simulink model "tekniska"  (R2018a)
settings: Solver=VariableStepAuto  StartTime=0.0  StopTime=3600  RelTol=1e-3
undefined symbols (not defined in the file): m, n
libraries: simulink x1
settings Model: Creator=wass  LastModifiedBy=wass

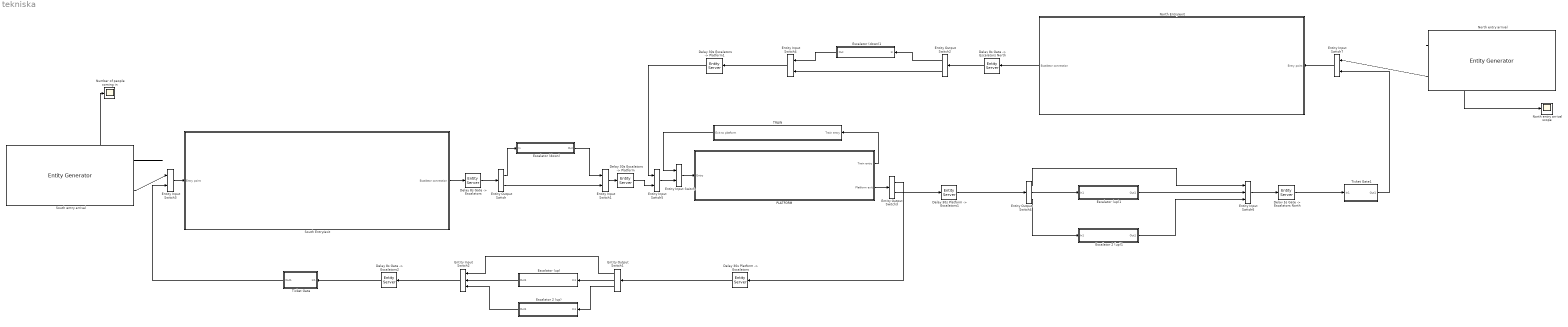
== system tekniska ==
  "Delay 30s Escalators -> Platform" : EntityServer  InputPortMessageModes=m  OutputPortMessageModes=m  Capacity=inf  ServiceTimeValue=30
  "Delay 30s Escalators -> Platform1" : EntityServer  InputPortMessageModes=m  OutputPortMessageModes=m  Capacity=inf  ServiceTimeValue=30
  "Delay 30s Platform -> Escalators" : EntityServer  InputPortMessageModes=m  OutputPortMessageModes=m  Capacity=inf  ServiceTimeValue=30
  "Delay 30s Platform -> Escalators1" : EntityServer  InputPortMessageModes=m  OutputPortMessageModes=m  Capacity=inf  ServiceTimeValue=30
  "Delay 5s Gate -> Escalators North" : EntityServer  InputPortMessageModes=m  OutputPortMessageModes=m  Capacity=inf  ServiceTimeValue=5
  "Delay 8s Gate -> Escalators" : EntityServer  InputPortMessageModes=m  OutputPortMessageModes=m  Capacity=inf  ServiceTimeValue=8
  "Delay 8s Gate -> Escalators North " : EntityServer  InputPortMessageModes=m  OutputPortMessageModes=m  Capacity=inf  ServiceTimeValue=5
  "Delay 8s Gate -> Escalators2" : EntityServer  InputPortMessageModes=m  OutputPortMessageModes=m  Capacity=inf  ServiceTimeValue=8
  Entity Input Switch{,1,3..5,7} (6 alike) : EntityInputSwitch  InputPortMessageModes=m,m  OutputPortMessageModes=m
  Entity Input Switch2 : EntityInputSwitch  InputPortMessageModes=m,m,m  OutputPortMessageModes=m  NumberInputPorts=3
      settings: InputPortMap=u1,u2,u3
  Entity Input Switch6 : EntityInputSwitch  InputPortMessageModes=m,m,m  OutputPortMessageModes=m  NumberInputPorts=3
      settings: InputPortMap=u1,u2,u3
  Entity Output Switch : EntityOutputSwitch  InputPortMessageModes=m  OutputPortMessageModes=m,m  SwitchingCriterion=Equiprobable  SwitchAttributeName=Attribute1
  Entity Output Switch1 : EntityOutputSwitch  InputPortMessageModes=m  OutputPortMessageModes=m,m,m  NumberOutputPorts=3  SwitchAttributeName=Attribute1
      settings: OutputPortMap=o0,o1,o2
  Entity Output Switch2 : EntityOutputSwitch  InputPortMessageModes=m  OutputPortMessageModes=m,m  SwitchingCriterion=Equiprobable  SwitchAttributeName=Attribute1
  Entity Output Switch3 : EntityOutputSwitch  InputPortMessageModes=m  OutputPortMessageModes=m,m  SwitchAttributeName=Attribute1
  Entity Output Switch4 : EntityOutputSwitch  InputPortMessageModes=m  OutputPortMessageModes=m,m,m  NumberOutputPorts=3  SwitchAttributeName=Attribute1
      settings: OutputPortMap=o0,o1,o2
  Escalator (down) : Subsystem
  Escalator (down)1 : Subsystem
  Escalator (up) : Subsystem
  Escalator (up)1 : Subsystem
  Escalator 2 (up) : Subsystem
  Escalator 2 (up)1 : Subsystem
  North Entry/exit : Subsystem
  North entry arrival : EntityGenerator  OutputPortMessageModes=n,m  TimeSource=MATLAB action  IntergenerationTimeAction=|  GenerateEntityAtSimulationStart=off  AttributeName=Incoming  AttributeInitialValue=2  NumberEntitiesDeparted=on  EntityType=Structured  EntityTypeName=Entity
      | wait_per_person = 10;
      | dt = exprnd(wait_per_person);
      settings: OutputPortMap=o0,o3
  North entry arrival scope : Scope
  Number of people coming in : Scope
  PLATFORM : Subsystem
  South Entry/exit : Subsystem
  South entry arrival : EntityGenerator  OutputPortMessageModes=n,m  TimeSource=MATLAB action  IntergenerationTimeAction=|  GenerateEntityAtSimulationStart=off  AttributeName=Incoming  AttributeInitialValue=2  NumberEntitiesDeparted=on  EntityType=Structured  EntityTypeName=Entity
      | wait_per_person = 5;
      | dt = exprnd(wait_per_person);
      settings: OutputPortMap=o0,o3
  TRAIN : Subsystem
  Ticket Gate : Subsystem
  Ticket Gate1 : Subsystem
  wires:
  TRAIN/1(Exit to platform) -> Entity Input Switch/1
  Escalator (up)/1(Out1) -> Entity Input Switch2/2
  Entity Input Switch/1 -> PLATFORM/1(Entry)
  South entry arrival/1 -> Number of people coming in/1
  Entity Output Switch1/3 -> Escalator 2 (up)/1(In1)
  PLATFORM/1(Train entry) -> TRAIN/1(Train entry)
  South Entry/exit/1(Escalator connection) -> "Delay 8s Gate -> Escalators"/1
  Escalator (down)/1(Out) -> Entity Input Switch1/1
  South entry arrival/2 -> Entity Input Switch3/1
  Entity Output Switch/1 -> Escalator (down)/1(In)
  Entity Output Switch1/2 -> Escalator (up)/1(In1)
  Entity Input Switch2/1 -> "Delay 8s Gate -> Escalators2"/1
  Entity Output Switch1/1 -> Entity Input Switch2/1
  Entity Input Switch1/1 -> "Delay 30s Escalators -> Platform"/1
  Escalator 2 (up)/1(Out1) -> Entity Input Switch2/3
  Entity Input Switch3/1 -> South Entry/exit/1(Entry point)
  Ticket Gate/1(Out1) -> Entity Input Switch3/2
  Entity Output Switch/2 -> Entity Input Switch1/2
  "Delay 8s Gate -> Escalators"/1 -> Entity Output Switch/1
  "Delay 8s Gate -> Escalators2"/1 -> Ticket Gate/1(In1)
  "Delay 30s Platform -> Escalators"/1 -> Entity Output Switch1/1
  Escalator (down)1/1(Out) -> Entity Input Switch4/1
  Entity Output Switch2/1 -> Escalator (down)1/1(In)
  Entity Output Switch2/2 -> Entity Input Switch4/2
  North Entry/exit/1(Escalator connection) -> "Delay 8s Gate -> Escalators North "/1
  "Delay 8s Gate -> Escalators North "/1 -> Entity Output Switch2/1
  Entity Input Switch4/1 -> "Delay 30s Escalators -> Platform1"/1
  "Delay 30s Escalators -> Platform"/1 -> Entity Input Switch5/2
  "Delay 30s Escalators -> Platform1"/1 -> Entity Input Switch5/1
  Entity Input Switch5/1 -> Entity Input Switch/2
  PLATFORM/2(Platform exit) -> Entity Output Switch3/1
  Entity Output Switch3/1 -> "Delay 30s Platform -> Escalators"/1
  Entity Output Switch3/2 -> "Delay 30s Platform -> Escalators1"/1
  Entity Input Switch6/1 -> "Delay 5s Gate -> Escalators North"/1
  Ticket Gate1/1(Out1) -> Entity Input Switch7/2
  Entity Output Switch4/2 -> Escalator (up)1/1(In1)
  Entity Output Switch4/3 -> Escalator 2 (up)1/1(In1)
  Escalator (up)1/1(Out1) -> Entity Input Switch6/2
  Escalator 2 (up)1/1(Out1) -> Entity Input Switch6/3
  Entity Output Switch4/1 -> Entity Input Switch6/1
  "Delay 30s Platform -> Escalators1"/1 -> Entity Output Switch4/1
  "Delay 5s Gate -> Escalators North"/1 -> Ticket Gate1/1(In1)
  Entity Input Switch7/1 -> North Entry/exit/1(Entry point)
  North entry arrival/1 -> North entry arrival scope/1
  North entry arrival/2 -> Entity Input Switch7/1

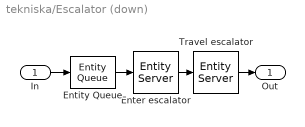
== system tekniska/Escalator (down) ==
  In : Inport
  Enter escalator : EntityServer  InputPortMessageModes=m  OutputPortMessageModes=m  Capacity=1  ServiceTimeValue=1
  Entity Queue : EntityQueue  InputPortMessageModes=m  OutputPortMessageModes=m  Capacity=inf
      settings: OutputPortMap=o5
  Travel escalator : EntityServer  InputPortMessageModes=m  OutputPortMessageModes=m  Capacity=inf  ServiceTimeValue=40
  Out : Outport
  wires:
  In/1 -> Entity Queue/1
  Enter escalator/1 -> Travel escalator/1
  Travel escalator/1 -> Out/1
  Entity Queue/1 -> Enter escalator/1

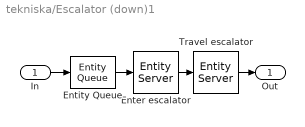
== system tekniska/Escalator (down)1 ==
  In : Inport
  Enter escalator : EntityServer  InputPortMessageModes=m  OutputPortMessageModes=m  Capacity=1  ServiceTimeValue=1
  Entity Queue : EntityQueue  InputPortMessageModes=m  OutputPortMessageModes=m  Capacity=inf
      settings: OutputPortMap=o5
  Travel escalator : EntityServer  InputPortMessageModes=m  OutputPortMessageModes=m  Capacity=inf  ServiceTimeValue=40
  Out : Outport
  wires:
  In/1 -> Entity Queue/1
  Enter escalator/1 -> Travel escalator/1
  Travel escalator/1 -> Out/1
  Entity Queue/1 -> Enter escalator/1

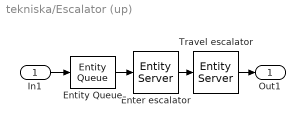
== system tekniska/Escalator (up) ==
  In1 : Inport
  Enter escalator : EntityServer  InputPortMessageModes=m  OutputPortMessageModes=m  Capacity=1  ServiceTimeValue=1
  Entity Queue : EntityQueue  InputPortMessageModes=m  OutputPortMessageModes=m  Capacity=inf
      settings: OutputPortMap=o5
  Travel escalator : EntityServer  InputPortMessageModes=m  OutputPortMessageModes=m  Capacity=inf  ServiceTimeValue=40
  Out1 : Outport
  wires:
  In1/1 -> Entity Queue/1
  Enter escalator/1 -> Travel escalator/1
  Travel escalator/1 -> Out1/1
  Entity Queue/1 -> Enter escalator/1

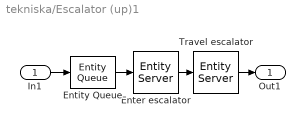
== system tekniska/Escalator (up)1 ==
  In1 : Inport
  Enter escalator : EntityServer  InputPortMessageModes=m  OutputPortMessageModes=m  Capacity=1  ServiceTimeValue=1
  Entity Queue : EntityQueue  InputPortMessageModes=m  OutputPortMessageModes=m  Capacity=inf
      settings: OutputPortMap=o5
  Travel escalator : EntityServer  InputPortMessageModes=m  OutputPortMessageModes=m  Capacity=inf  ServiceTimeValue=40
  Out1 : Outport
  wires:
  In1/1 -> Entity Queue/1
  Enter escalator/1 -> Travel escalator/1
  Travel escalator/1 -> Out1/1
  Entity Queue/1 -> Enter escalator/1

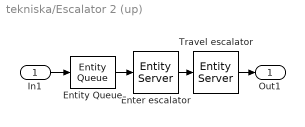
== system tekniska/Escalator 2 (up) ==
  In1 : Inport
  Enter escalator : EntityServer  InputPortMessageModes=m  OutputPortMessageModes=m  Capacity=1  ServiceTimeValue=1
  Entity Queue : EntityQueue  InputPortMessageModes=m  OutputPortMessageModes=m  Capacity=inf
      settings: OutputPortMap=o5
  Travel escalator : EntityServer  InputPortMessageModes=m  OutputPortMessageModes=m  Capacity=inf  ServiceTimeValue=40
  Out1 : Outport
  wires:
  In1/1 -> Entity Queue/1
  Enter escalator/1 -> Travel escalator/1
  Travel escalator/1 -> Out1/1
  Entity Queue/1 -> Enter escalator/1

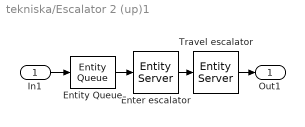
== system tekniska/Escalator 2 (up)1 ==
  In1 : Inport
  Enter escalator : EntityServer  InputPortMessageModes=m  OutputPortMessageModes=m  Capacity=1  ServiceTimeValue=1
  Entity Queue : EntityQueue  InputPortMessageModes=m  OutputPortMessageModes=m  Capacity=inf
      settings: OutputPortMap=o5
  Travel escalator : EntityServer  InputPortMessageModes=m  OutputPortMessageModes=m  Capacity=inf  ServiceTimeValue=40
  Out1 : Outport
  wires:
  In1/1 -> Entity Queue/1
  Enter escalator/1 -> Travel escalator/1
  Travel escalator/1 -> Out1/1
  Entity Queue/1 -> Enter escalator/1

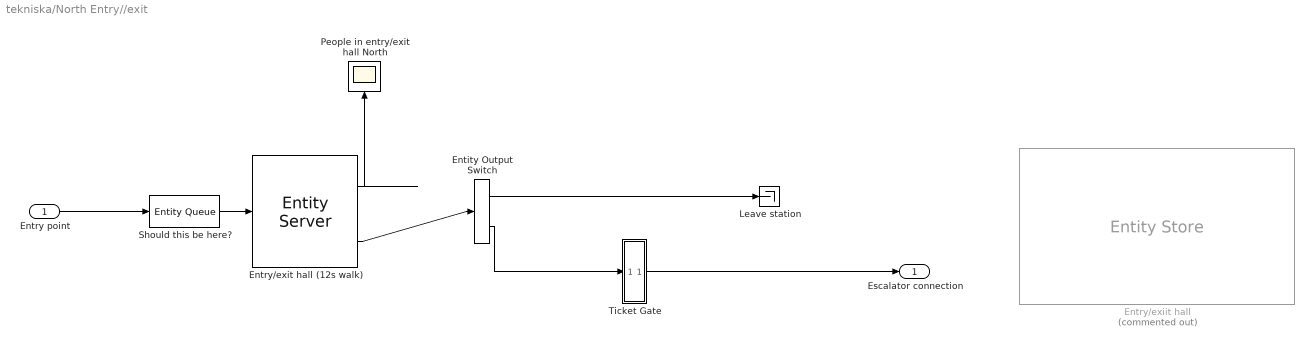
== system tekniska/North Entry//exit ==
  Entry point : Inport
  Entity Output Switch : EntityOutputSwitch  InputPortMessageModes=m  OutputPortMessageModes=m,m  SwitchingCriterion=From attribute  SwitchAttributeName=Incoming
  Entry/exiit hall : EntityStore  Commented=on  InputPortMessageModes=m  OutputPortMessageModes=n,m  Capacity=100  NumberEntitiesInBlock=on
      settings: OutputPortMap=o1,o4
  Entry/exit hall (12s walk) : EntityServer  InputPortMessageModes=m  OutputPortMessageModes=n,m  Capacity=100  ServiceTimeValue=12  NumberEntitiesInBlock=on
      settings: OutputPortMap=o1,o9
  Leave station : Terminator
  "People in entry/exit hall North " : Scope
  Should this be here? : EntityQueue  InputPortMessageModes=m  OutputPortMessageModes=m  Capacity=inf
      settings: OutputPortMap=o5
  Ticket Gate : Subsystem
  Escalator connection : Outport
  wires:
  Entry/exit hall (12s walk)/1 -> "People in entry/exit hall North "/1
  Entry/exit hall (12s walk)/2 -> Entity Output Switch/1
  Entry point/1 -> Should this be here?/1
  Entity Output Switch/1 -> Leave station/1
  Entity Output Switch/2 -> Ticket Gate/1(In1)
  Should this be here?/1 -> Entry/exit hall (12s walk)/1
  Ticket Gate/1(Out1) -> Escalator connection/1

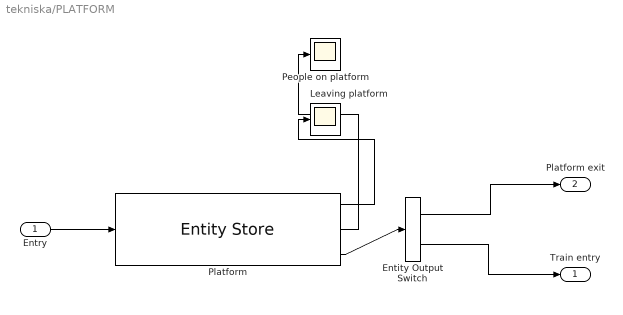
== system tekniska/PLATFORM ==
  Entry : Inport
  Entity Output Switch : EntityOutputSwitch  InputPortMessageModes=m  OutputPortMessageModes=m,m  SwitchingCriterion=From attribute  SwitchAttributeName=Incoming
  "Leaving platform " : Scope
  People on platform : Scope
  "Platform " : EntityStore  InputPortMessageModes=m  OutputPortMessageModes=n,n,m  Capacity=500  NumberEntitiesDeparted=on  NumberEntitiesInBlock=on
      settings: OutputPortMap=o0,o1,o4
  Train entry : Outport
  Platform exit : Outport  Port=2
  wires:
  "Platform "/2 -> People on platform/1
  "Platform "/1 -> "Leaving platform "/1
  Entry/1 -> "Platform "/1
  "Platform "/3 -> Entity Output Switch/1
  Entity Output Switch/1 -> Platform exit/1
  Entity Output Switch/2 -> Train entry/1

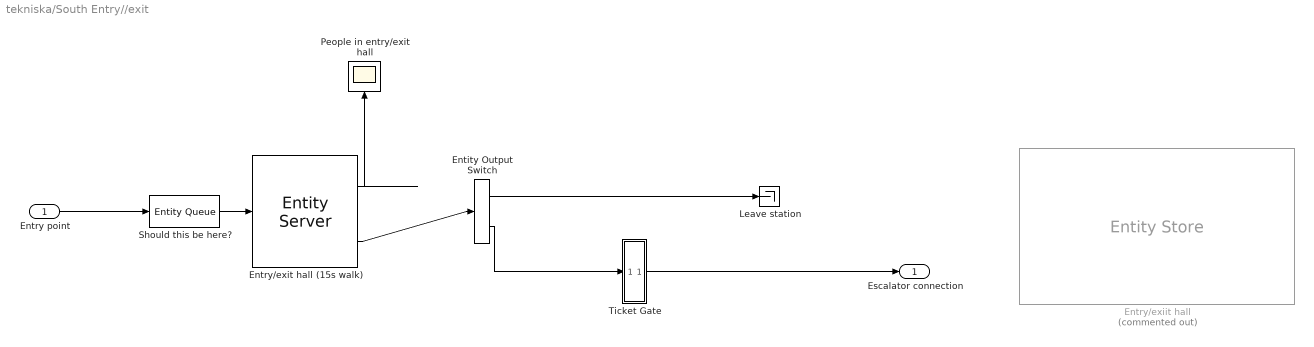
== system tekniska/South Entry//exit ==
  Entry point : Inport
  Entity Output Switch : EntityOutputSwitch  InputPortMessageModes=m  OutputPortMessageModes=m,m  SwitchingCriterion=From attribute  SwitchAttributeName=Incoming
  Entry/exiit hall : EntityStore  Commented=on  InputPortMessageModes=m  OutputPortMessageModes=n,m  Capacity=100  NumberEntitiesInBlock=on
      settings: OutputPortMap=o1,o4
  Entry/exit hall (15s walk) : EntityServer  InputPortMessageModes=m  OutputPortMessageModes=n,m  Capacity=100  ServiceTimeValue=15  NumberEntitiesInBlock=on
      settings: OutputPortMap=o1,o9
  Leave station : Terminator
  "People in entry/exit hall " : Scope
  Should this be here? : EntityQueue  InputPortMessageModes=m  OutputPortMessageModes=m  Capacity=inf
      settings: OutputPortMap=o5
  Ticket Gate : Subsystem
  Escalator connection : Outport
  wires:
  Entry/exit hall (15s walk)/1 -> "People in entry/exit hall "/1
  Entry/exit hall (15s walk)/2 -> Entity Output Switch/1
  Entry point/1 -> Should this be here?/1
  Entity Output Switch/1 -> Leave station/1
  Entity Output Switch/2 -> Ticket Gate/1(In1)
  Should this be here?/1 -> Entry/exit hall (15s walk)/1
  Ticket Gate/1(Out1) -> Escalator connection/1

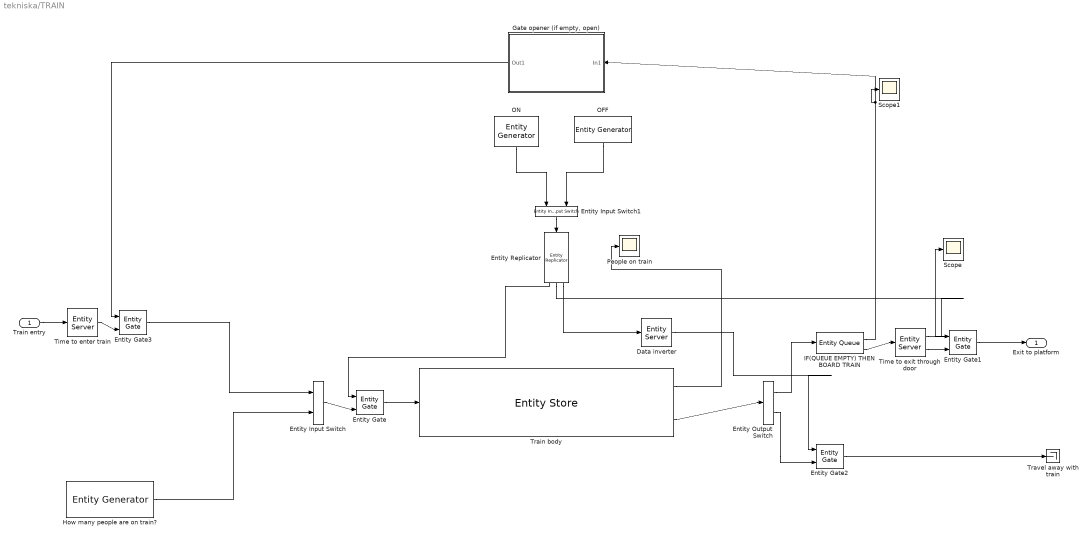
== system tekniska/TRAIN ==
  Train entry : Inport
  Data inverter : EntityServer  InputPortMessageModes=m  OutputPortMessageModes=m  Capacity=inf  ServiceTimeValue=0  EntryAction=entity = 1 - entity;
  Entity Input Switch : EntityInputSwitch  InputPortMessageModes=m,m  OutputPortMessageModes=m
  Entity Input Switch1 : EntityInputSwitch  InputPortMessageModes=m,m  OutputPortMessageModes=m
  Entity Output Switch : EntityOutputSwitch  InputPortMessageModes=m  OutputPortMessageModes=m,m  SwitchingCriterion=From attribute  SwitchAttributeName=Incoming
  Entity Gate{,1..3} (4 alike) : EntityGate  InputPortMessageModes=m,m  OutputPortMessageModes=m
  Entity Replicator : EntityReplicator  InputPortMessageModes=m  OutputPortMessageModes=m,m,m  NumberReplicas=2  HoldOriginalEntityUntilAllReplicasDepart=on
      settings: OutputPortMap=o0,o1,o2
  "Gate opener (if empty, open)" : Subsystem
  "How many people are on train? " : EntityGenerator  OutputPortMessageModes=m  TimeSource=MATLAB action  IntergenerationTimeAction=|  GenerateEntityAtSimulationStart=off  GenerateAction=|  AttributeName=Incoming  EntityType=Structured  EntityTypeName=Entity
      IntergenerationTimeAction=|
      | persistent entity_number
      | 
      | people_per_wave = 100;
      | train_periodicity = 6*60;
      | 
      | if isempty(entity_number)
      |     entity_number = 1;
      | end
      | 
      | if entity_number == 1
      |     dt = train_periodicity - 60;
      | 
      | elseif mod(entity_number, people_per_wave) == 1
      |     dt = train_periodicity;
      | else
      |     dt = 0;
      | end
      |     
      |         
      |     
      |     
      | entity_number = entity_number + 1;
      GenerateAction=|
      | prob_incoming = 0.1;
      | 
      | entity.Incoming = 1 + (rand() > prob_incoming);
  IF(QUEUE EMPTY) THEN BOARD TRAIN : EntityQueue  InputPortMessageModes=m  OutputPortMessageModes=n,m  NumberEntitiesInBlock=on
      settings: OutputPortMap=o1,o5
  OFF : EntityGenerator  OutputPortMessageModes=m  Period=6*60  IntergenerationTimeAction=dt = 5;  GenerateEntityAtSimulationStart=off  AttributeName=entity  AttributeInitialValue=0  EntityTypeName=Entity
  ON : EntityGenerator  OutputPortMessageModes=m  TimeSource=MATLAB action  Period=5  IntergenerationTimeAction=|  GenerateEntityAtSimulationStart=off  AttributeName=entity  EntityTypeName=Entity  DataInitialValue=1
      | persistent first
      | if isempty(first)
      |     first = true;
      |     dt = 5*60; 
      | else
      |     dt = 6*60;
      | end
  People on train : Scope
  Scope : Scope
  Scope1 : Scope
  Time to exit through door : EntityServer  InputPortMessageModes=m  OutputPortMessageModes=n,m  Capacity=42  ServiceTimeValue=1  NumberEntitiesInBlock=on
      settings: OutputPortMap=o1,o9
  Time to enter train : EntityServer  InputPortMessageModes=m  OutputPortMessageModes=m  Capacity=42  ServiceTimeValue=1  ServiceTimeAction=|
      | % Time to enter train should depend on how
      | % many people are leaving / staying on the train
      | dt = 1;
  Train body : EntityStore  InputPortMessageModes=m  OutputPortMessageModes=n,m  Capacity=200  NumberEntitiesInBlock=on
      settings: OutputPortMap=o1,o4
  Travel away with train : Terminator
  Exit to platform : Outport
  wires:
  ON/1 -> Entity Input Switch1/1
  OFF/1 -> Entity Input Switch1/2
  "How many people are on train? "/1 -> Entity Input Switch/2
  Entity Gate3/1 -> Entity Input Switch/1
  Entity Gate1/1 -> Exit to platform/1
  Entity Gate/1 -> Train body/1
  Entity Input Switch/1 -> Entity Gate/2
  Entity Input Switch1/1 -> Entity Replicator/1
  Entity Replicator/1 -> Entity Gate/1
  Entity Replicator/2 -> Entity Gate1/1
  Train body/2 -> Entity Output Switch/1
  Entity Output Switch/2 -> Entity Gate2/2
  Entity Replicator/3 -> Data inverter/1
  Data inverter/1 -> Entity Gate2/1
  Entity Gate2/1 -> Travel away with train/1
  Time to exit through door/2 -> Entity Gate1/2
  Entity Output Switch/1 -> IF(QUEUE EMPTY) THEN BOARD TRAIN/1
  IF(QUEUE EMPTY) THEN BOARD TRAIN/2 -> Time to exit through door/1
  Time to exit through door/1 -> Scope/1
  Train body/1 -> People on train/1
  IF(QUEUE EMPTY) THEN BOARD TRAIN/1 -> Scope1/1, "Gate opener (if empty, open)"/1(In1)
  "Gate opener (if empty, open)"/1(Out1) -> Entity Gate3/1
  Train entry/1 -> Time to enter train/1
  Time to enter train/1 -> Entity Gate3/2

== system tekniska/Ticket Gate ==
  In1 : Inport
  Ticket Gates : EntityServer  InputPortMessageModes=m  OutputPortMessageModes=m  Capacity=4  ServiceTimeValue=2
  Ticket gate queue : EntityQueue  InputPortMessageModes=m  OutputPortMessageModes=m  Capacity=inf
      settings: OutputPortMap=o5
  Out1 : Outport
  wires:
  Ticket gate queue/1 -> Ticket Gates/1
  Ticket Gates/1 -> Out1/1
  In1/1 -> Ticket gate queue/1

== system tekniska/Ticket Gate1 ==
  In1 : Inport
  Ticket Gates : EntityServer  InputPortMessageModes=m  OutputPortMessageModes=m  Capacity=4  ServiceTimeValue=2
  Ticket gate queue : EntityQueue  InputPortMessageModes=m  OutputPortMessageModes=m  Capacity=inf
      settings: OutputPortMap=o5
  Out1 : Outport
  wires:
  Ticket gate queue/1 -> Ticket Gates/1
  Ticket Gates/1 -> Out1/1
  In1/1 -> Ticket gate queue/1

== system tekniska/North Entry//exit/Ticket Gate ==
  In1 : Inport
  Ticket Gates : EntityServer  InputPortMessageModes=m  OutputPortMessageModes=m  ServiceTimeValue=4
  Ticket gate queue : EntityQueue  InputPortMessageModes=m  OutputPortMessageModes=m  Capacity=inf
      settings: OutputPortMap=o5
  Out1 : Outport
  wires:
  Ticket gate queue/1 -> Ticket Gates/1
  Ticket Gates/1 -> Out1/1
  In1/1 -> Ticket gate queue/1

== system tekniska/South Entry//exit/Ticket Gate ==
  In1 : Inport
  Ticket Gates : EntityServer  InputPortMessageModes=m  OutputPortMessageModes=m  ServiceTimeValue=4
  Ticket gate queue : EntityQueue  InputPortMessageModes=m  OutputPortMessageModes=m  Capacity=inf
      settings: OutputPortMap=o5
  Out1 : Outport
  wires:
  Ticket gate queue/1 -> Ticket Gates/1
  Ticket Gates/1 -> Out1/1
  In1/1 -> Ticket gate queue/1

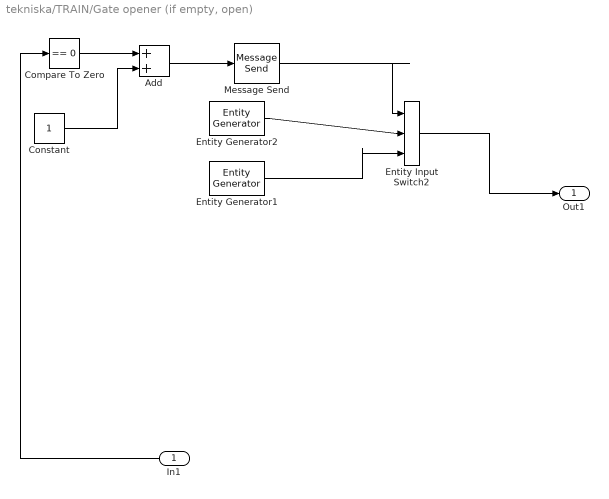
== system tekniska/TRAIN/Gate opener (if empty, open) ==
  In1 : Inport
  Add : Sum
  Compare To Zero : simulink/Logic and Bit Operations/Compare To Zero  relop===  OutDataTypeStr=uint8
  Constant : Constant
  Entity Input Switch2 : EntityInputSwitch  InputPortMessageModes=m,m,m  OutputPortMessageModes=m  ActivePortSelection=Switch  SwitchingCriterion=From control port
      settings: InputPortMap=u0,u1,u2
  Entity Generator1 : EntityGenerator  OutputPortMessageModes=m  Period=0.1  AttributeName=entity  EntityTypeName=asd  DataInitialValue=1
  Entity Generator2 : EntityGenerator  OutputPortMessageModes=m  Period=0.1  AttributeName=entity  AttributeInitialValue=0  EntityTypeName=Entity
  Message Send : MessageSend  OutputPortMessageModes=m
      settings: InputPortMap=u1
  Out1 : Outport
  wires:
  Compare To Zero/1 -> Add/1
  In1/1 -> Compare To Zero/1
  Message Send/1 -> Entity Input Switch2/1
  Constant/1 -> Add/2
  Entity Input Switch2/1 -> Out1/1
  Entity Generator2/1 -> Entity Input Switch2/2
  Entity Generator1/1 -> Entity Input Switch2/3
  Add/1 -> Message Send/1
